simulink model "YawModel_R2"  (R2013a)
settings: Solver=ode45  StartTime=0.0  StopTime=10  RelTol=1e-3
values from neighbouring files (symbols this model uses):
  D = 4.45306861536e-07    [Parameters.mat]
  I_Psi = 0.236966962973    [Parameters.mat]
  J = 8e-08    [Parameters.mat]
  Kp_Yaw = K    [Yaw_PID.m]
  Kw = 501.513336009    [Parameters.mat]
  Motor_TimeConstant = 0.07    [Parameters.mat]
  omega_0 = 520    [Yaw_PID.m]
  Speed_yIntercept = -347.939581678    [Parameters.mat]
  T_I = (1/(2*v))*((imag(DCL_Pole_1)/2)-(real(DCL_Pole_1)*v))    [Pitch_Roll_Controller_PID.m]    (also in Yaw_PID.m)
libraries: simulink x3
settings Model: Creator=Ross  LastModifiedBy=Ross

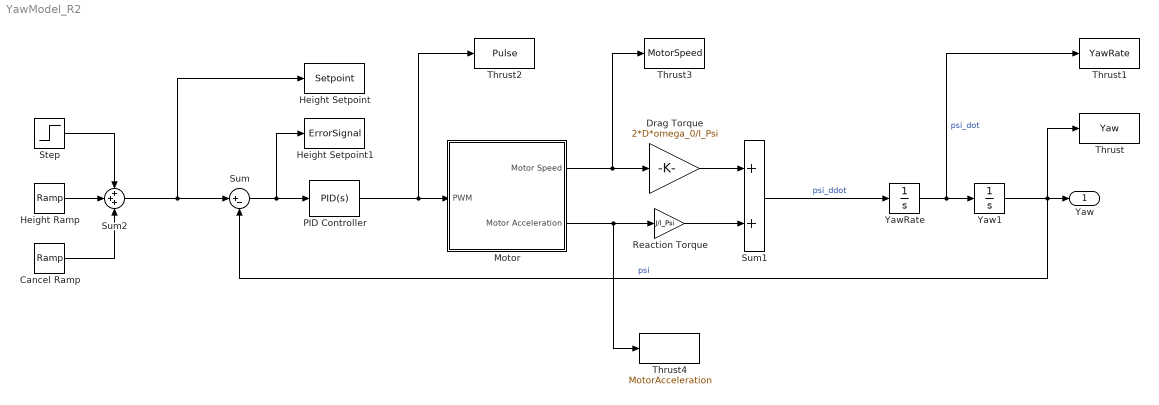
== system YawModel_R2 ==
  Cancel Ramp : simulink/Sources/Ramp  slope=-1  start=2  X0=0
  Drag Torque : Gain  Gain=2*D*omega_0/I_Psi
  Height Ramp : simulink/Sources/Ramp  slope=1  start=1  X0=0
  Height Setpoint : ToWorkspace  VariableName=Setpoint  SampleTime=-1  SaveFormat=Timeseries
  Height Setpoint1 : ToWorkspace  VariableName=ErrorSignal  SampleTime=-1  SaveFormat=Timeseries
  Motor : Subsystem
  PID Controller : simulink/Continuous/PID Controller  Controller=PID  TimeDomain=Continuous-time  SampleTime=1  IntegratorMethod=Forward Euler  FilterMethod=Forward Euler  Form=Ideal  P=Kp_Yaw  I=1/T_I  D=T_I/4  N=100  InitialConditionSource=internal  InitialConditionForIntegrator=0  InitialConditionForFilter=0  ExternalReset=none  LimitOutput=off  UpperSaturationLimit=2  LowerSaturationLimit=0  LinearizeAsGain=on  AntiWindupMode=clamping  Kb=1  TrackingMode=off  Kt=1  PParamMin=[]  PParamMax=[]  IParamMin=[]  IParamMax=[]  DParamMin=[]  DParamMax=[]  NParamMin=[]  NParamMax=[]  KbParamMin=[]  KbParamMax=[]  KtParamMin=[]  KtParamMax=[]  POutMin=[]  POutMax=[]  IOutMin=[]  IOutMax=[]  DOutMin=[]  DOutMax=[]  NOutMin=[]  NOutMax=[]  KbOutMin=[]  KbOutMax=[]  KtOutMin=[]  KtOutMax=[]  IntegratorOutMin=[]  IntegratorOutMax=[]  FilterOutMin=[]  FilterOutMax=[]  SumOutMin=[]  SumOutMax=[]  SumI1OutMin=[]  SumI1OutMax=[]  SumI2OutMin=[]  SumI2OutMax=[]  SumI3OutMin=[]  SumI3OutMax=[]  SumDOutMin=[]  SumDOutMax=[]  SaturationOutMin=[]  SaturationOutMax=[]  IntegratorContinuousStateAttributes=''  IntegratorStateMustResolveToSignalObject=off  IntegratorRTWStateStorageClass=Auto  FilterContinuousStateAttributes=''  FilterStateMustResolveToSignalObject=off  FilterRTWStateStorageClass=Auto
  Reaction Torque : Gain  Gain=J/I_Psi
  Step : Step  Time=3  SampleTime=0
  Sum : Sum  Inputs=|+-
  Sum1 : Sum
  Sum2 : Sum  Inputs=+++
  Thrust : ToWorkspace  VariableName=Yaw  SampleTime=-1  SaveFormat=Timeseries
  Thrust1 : ToWorkspace  VariableName=YawRate  SampleTime=-1  SaveFormat=Timeseries
  Thrust2 : ToWorkspace  VariableName=Pulse  SampleTime=-1  SaveFormat=Timeseries
  Thrust3 : ToWorkspace  VariableName=MotorSpeed  SampleTime=-1  SaveFormat=Timeseries
  Thrust4 : ToWorkspace  VariableName=MotorAcceleration  SampleTime=-1  SaveFormat=Timeseries
  Yaw1 : Integrator  LowerSaturationLimit=0
  YawRate : Integrator
  Yaw : Outport
  wires:
  Yaw1/1 -> Sum/2, Thrust/1, Yaw/1  "psi"
  YawRate/1 -> Thrust1/1, Yaw1/1  "psi_dot"
  Sum1/1 -> YawRate/1  "psi_ddot"
  Motor/2(Motor Acceleration) -> Thrust4/1, Reaction Torque/1
  Drag Torque/1 -> Sum1/1
  Reaction Torque/1 -> Sum1/2
  PID Controller/1 -> Thrust2/1, Motor/1(PWM)
  Step/1 -> Sum2/1
  Height Ramp/1 -> Sum2/2
  Cancel Ramp/1 -> Sum2/3
  Sum2/1 -> Height Setpoint/1, Sum/1
  Sum/1 -> Height Setpoint1/1, PID Controller/1
  Motor/1(Motor Speed) -> Drag Torque/1, Thrust3/1

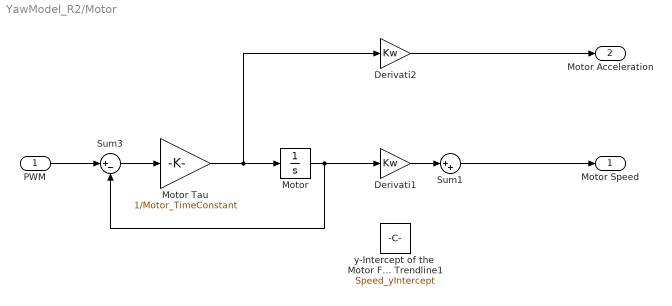
== system YawModel_R2/Motor ==
  PWM : Inport
  Derivati1 : Gain  Gain=Kw
  Derivati2 : Gain  Gain=Kw
  Motor : Integrator
  Motor Tau : Gain  Gain=1/Motor_TimeConstant
  Sum1 : Sum  Inputs=|++
  Sum3 : Sum  Inputs=|+-
  y-Intercept of the  Motor Forc Trendline1 : Constant  Value=Speed_yIntercept
  Motor Speed : Outport
  Motor Acceleration : Outport  Port=2
  wires:
  Motor Tau/1 -> Derivati2/1, Motor/1
  Motor/1 -> Derivati1/1, Sum3/2
  PWM/1 -> Sum3/1
  Sum3/1 -> Motor Tau/1
  Derivati1/1 -> Sum1/1
  Sum1/1 -> Motor Speed/1
  Derivati2/1 -> Motor Acceleration/1
